simulink model "simulink_problem_3_5_148_14"  (R2014a)
settings: Solver=ode45  SolverMode=SingleTasking  StartTime=0.0  StopTime=10.0  RelTol=1e-3
settings Model: CovMetricSettings=dwe  CovHtmlReporting=off  covSaveCumulativeToWorkspaceVar=off  CovSaveSingleToWorkspaceVar=off  CovExternalEMLEnable=on  CovSFcnEnable=on  Creator=ghost  LastModifiedBy=ghost
settings DataIOCC: LimitDataPoints=off  SaveFormat=StructureWithTime
settings DebuggingCC: MergeDetectMultiDrivingBlocksExec=error  SolverPrmCheckMsg=none  FrameProcessingCompatibilityMsg=error  SFUnexpectedBacktrackingDiag=error  SFNoUnconditionalDefaultTransitionDiag=error
settings HardwareCC: ProdBitPerPointer=64  ProdLargestAtomicFloat=Float  ProdIntDivRoundTo=Zero  ProdEndianess=LittleEndian  ProdHWDeviceType=Specified
settings ModelReferenceCC: PropagateSignalLabelsOutOfModel=on
settings GRTTargetCC: TargetLangStandard=C99 (ISO)  GeneratePreprocessorConditionals=Use local settings

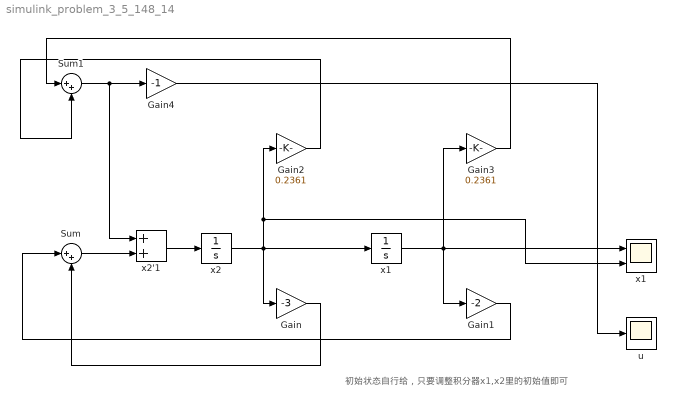
== system simulink_problem_3_5_148_14 ==
  note: 初始状态自行给，只要调整积分器x1,x2里的初始值即可
  Gain : Gain  Gain=-3
  Gain1 : Gain  Gain=-2
  Gain2 : Gain  Gain=0.2361
  Gain3 : Gain  Gain=0.2361
  Gain4 : Gain  Gain=-1
  Sum : Sum  Inputs=|++
  Sum1 : Sum  Inputs=|++
  u : Scope
      settings: TimeRange=auto  MaxDataPoints=5000  SaveToWorkspace=off  SaveName=ScopeData2  YMin=-28.39005  YMax=5.51043  SampleTime=-1
  x1 : Scope  NumInputPorts=2
      settings: TimeRange=auto  MaxDataPoints=5000  SaveToWorkspace=off  SaveName=ScopeData  YMin=-3.75319~-5  YMax=6.70799~5  SampleTime=-1
  "x1 " : Integrator  InitialCondition=5
  "x2 " : Integrator  InitialCondition=5
  x2'1 : Sum
  wires:
  "x2 "/1 -> "x1 "/1, x1/2, Gain2/1, Gain/1
  Gain/1 -> Sum/2
  "x1 "/1 -> Gain3/1, x1/1, Gain1/1
  Gain1/1 -> Sum/1
  x2'1/1 -> "x2 "/1
  Sum/1 -> x2'1/2
  Gain2/1 -> Sum1/2
  Gain3/1 -> Sum1/1
  Sum1/1 -> Gain4/1, x2'1/1
  Gain4/1 -> u/1
